simulink model "satellite_sim"  (Simulink 7.5)
settings: Solver=ode45  StartTime=0.0  StopTime=10000  RelTol=1e-3
undefined symbols (not defined in the file or in its folder): drawSatellite
libraries: simulink x1
settings Model: Creator=beard  LastModifiedBy=rwb5
settings OptimizationCC: InitFltsAndDblsToZero=on
settings DebuggingCC: StrictBusMsg=Warning

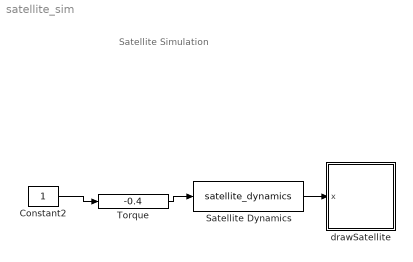
== system satellite_sim ==
  note: Satellite Simulation
  Constant2 : Constant  OutDataType=sfix(16)  OutScaling=2^0
  Satellite Dynamics : S-Function  FunctionName=satellite_dynamics  Parameters=AP  EnableBusSupport=off
  Torque : simulink/Math Operations/Slider Gain  SystemSampleTime=-1  low=-10  gain=-0.4  high=10
  drawSatellite : Subsystem
      mask init:
      | % drawing parameters
      | L = 1;
      | w = .3;
      mask Display: image(imread('tv.jpg'))
  wires:
  Constant2/1 -> Torque/1
  Satellite Dynamics/1 -> drawSatellite/1(x)
  Torque/1 -> Satellite Dynamics/1

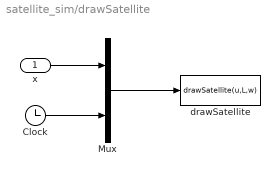
== system satellite_sim/drawSatellite ==
  x : Inport
  Clock : Clock
      settings: Decimation=10
  Mux : Mux  Inputs=2
  drawSatellite : MATLABFcn  MATLABFcn=drawSatellite(u,L,w)  OutputDimensions=0  SampleTime=0.1
  wires:
  Mux/1 -> drawSatellite/1
  x/1 -> Mux/1
  Clock/1 -> Mux/2
